simulink model "q2w2"  (R2024b)
settings: Solver=VariableStepAuto  StartTime=0.0  StopTime=10.0  RelTol=1e-3

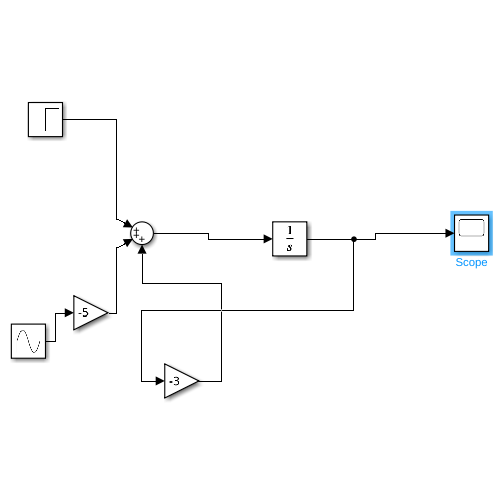
[thumbnail: Simulink's stored preview of the top-level diagram]
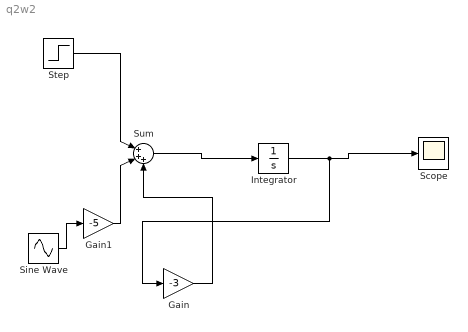
== system q2w2 ==
  Gain : Gain  Gain=-3
  Gain1 : Gain  Gain=-5
  Integrator : Integrator
  Scope : Scope
  Sine Wave : Sin  SampleTime=0
  Step : Step  SampleTime=0
  Sum : Sum  Inputs=|+++
  wires:
  Integrator/1 -> Gain/1, Scope/1
  Sum/1 -> Integrator/1
  Gain1/1 -> Sum/2
  Sine Wave/1 -> Gain1/1
  Step/1 -> Sum/1
  Gain/1 -> Sum/3
